simulink model "VK"  (R2022b)
settings: Solver=ode1  StartTime=0.0  StopTime=240  FixedStep=0.01  RelTol=1e-3
undefined symbols (not defined in the file): F, Light, MIL, Newton, Raphson, sigbuilder_block
libraries: simulink x3, aerolibwind2 x2, aerolibutil x1, sharedtransform x1
settings Model: Creator=jmira  LastModifiedBy=armando
settings DebuggingCC: UnconnectedInputMsg=warning  UnconnectedOutputMsg=warning  UnconnectedLineMsg=warning
settings ModelReferenceCC: EnableRefExpFcnMdlSchedulingChecks=on
settings RTWCC: DLArmComputeVersion=19.05

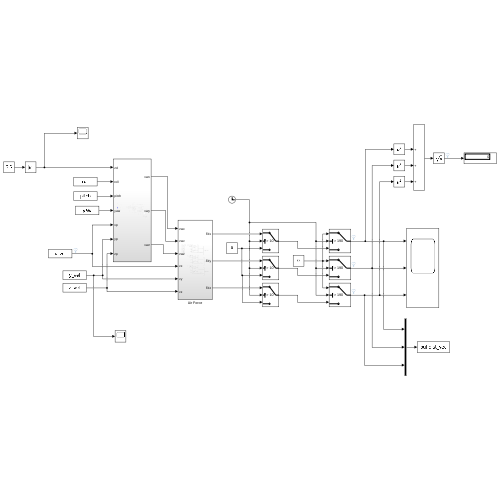
[thumbnail: Simulink's stored preview of the top-level diagram]
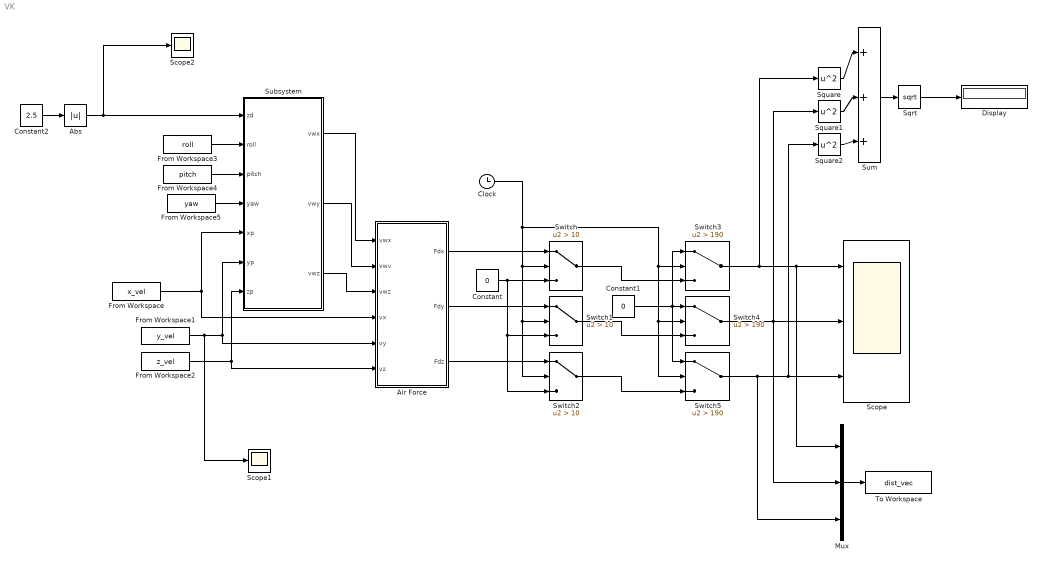
== system VK ==
  Abs : Abs  SaturateOnIntegerOverflow=off
  Air Force : Subsystem
  Clock : Clock
  Constant : Constant  Value=0
  Constant1 : Constant  Value=0
  Constant2 : Constant  Value=2.5
  Display : Display
  From Workspace : FromWorkspace  VariableName=x_vel  SampleTime=0.01
  From Workspace1 : FromWorkspace  VariableName=y_vel  SampleTime=0.01
  From Workspace2 : FromWorkspace  VariableName=z_vel  SampleTime=0.01
  From Workspace3 : FromWorkspace  VariableName=roll  SampleTime=0.01
  From Workspace4 : FromWorkspace  VariableName=pitch  SampleTime=0.01
  From Workspace5 : FromWorkspace  VariableName=yaw  SampleTime=0.01
  Mux : Mux  Inputs=3
  Scope : Scope  NumInputPorts=3
  Scope1 : Scope
  Scope2 : Scope
  Sqrt : Sqrt
  Square : Math  Operator=square
  Square1 : Math  Operator=square
  Square2 : Math  Operator=square
  Subsystem : Subsystem
  Sum : Sum  Inputs=|+++
  Switch : Switch  Criteria=u2 > Threshold  Threshold=10  SaturateOnIntegerOverflow=off  InputSameDT=off
  Switch1 : Switch  Criteria=u2 > Threshold  Threshold=10  SaturateOnIntegerOverflow=off  InputSameDT=off
  Switch2 : Switch  Criteria=u2 > Threshold  Threshold=10  SaturateOnIntegerOverflow=off  InputSameDT=off
  Switch3 : Switch  Criteria=u2 > Threshold  Threshold=190  SaturateOnIntegerOverflow=off  InputSameDT=off
  Switch4 : Switch  Criteria=u2 > Threshold  Threshold=190  SaturateOnIntegerOverflow=off  InputSameDT=off
  Switch5 : Switch  Criteria=u2 > Threshold  Threshold=190  SaturateOnIntegerOverflow=off  InputSameDT=off
  To Workspace : ToWorkspace  VariableName=dist_vec  SampleTime=-1
      settings: Save2DSignal=2-D array (concatenate along first dimension)
  wires:
  Abs/1 -> Scope2/1, Subsystem/1(zd)
  Subsystem/1(vwx) -> Air Force/1(vwx)
  From Workspace/1 -> Air Force/4(vx), Subsystem/5(xp)
  Subsystem/3(vwz) -> Air Force/3(vwz)
  From Workspace1/1 -> Scope1/1, Air Force/5(vy), Subsystem/6(yp)
  Subsystem/2(vwy) -> Air Force/2(vwv)
  From Workspace2/1 -> Air Force/6(vz), Subsystem/7(zp)
  From Workspace3/1 -> Subsystem/2(roll)
  From Workspace4/1 -> Subsystem/3(pitch)
  From Workspace5/1 -> Subsystem/4(yaw)
  Mux/1 -> To Workspace/1
  Air Force/1(Fdx) -> Switch/1
  Clock/1 -> Switch5/2, Switch4/2, Switch3/2, Switch2/2, Switch1/2, Switch/2
  Constant/1 -> Switch2/3, Switch1/3, Switch/3
  Air Force/2(Fdy) -> Switch1/1
  Air Force/3(Fdz) -> Switch2/1
  Switch/1 -> Switch3/3
  Constant1/1 -> Switch5/1, Switch3/1, Switch4/1
  Switch1/1 -> Switch4/3
  Switch2/1 -> Switch5/3
  Switch3/1 -> Square/1, Mux/1, Scope/1
  Switch4/1 -> Square1/1, Mux/2, Scope/2
  Switch5/1 -> Mux/3, Square2/1, Scope/3
  Constant2/1 -> Abs/1
  Square/1 -> Sum/1
  Square2/1 -> Sum/3
  Square1/1 -> Sum/2
  Sum/1 -> Sqrt/1
  Sqrt/1 -> Display/1

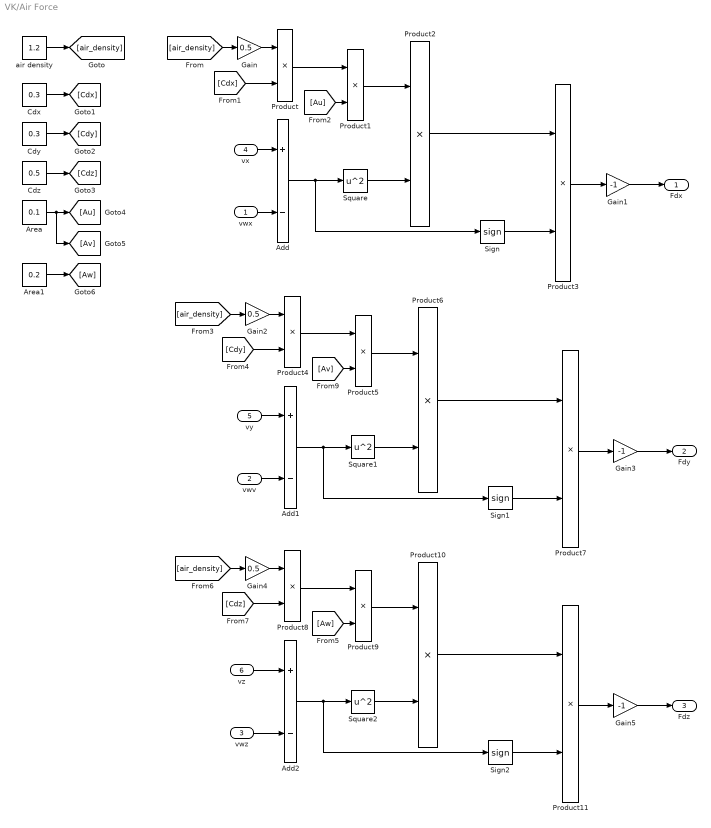
== system VK/Air Force ==
  vwx : Inport
  vwv : Inport  Port=2
  vwz : Inport  Port=3
  vx : Inport  Port=4
  vy : Inport  Port=5
  vz : Inport  Port=6
  Add : Sum  Inputs=+-
  Add1 : Sum  Inputs=+-
  Add2 : Sum  Inputs=+-
  Area : Constant  Value=0.1
  Area1 : Constant  Value=0.2
  Cdx : Constant  Value=0.3
  Cdy : Constant  Value=0.3
  Cdz : Constant  Value=0.5
  Gain : Gain  Gain=0.5
  Gain1 : Gain  Gain=-1
  Gain2 : Gain  Gain=0.5
  Gain3 : Gain  Gain=-1
  Gain4 : Gain  Gain=0.5
  Gain5 : Gain  Gain=-1
  Product{,1..11} (12 alike) : Product
  Sign : Signum
  Sign1 : Signum
  Sign2 : Signum
  Square : Math  Operator=square
  Square1 : Math  Operator=square
  Square2 : Math  Operator=square
  air density : Constant  Value=1.2
  Fdx : Outport
  Fdy : Outport  Port=2
  Fdz : Outport  Port=3
  wires:
  air density/1 -> [air_density]
  [air_density] -> Gain/1
  Cdx/1 -> [Cdx]
  Cdy/1 -> [Cdy]
  Cdz/1 -> [Cdz]
  Gain/1 -> Product/1
  [Cdx] -> Product/2
  Area/1 -> [Av], [Au]
  Product/1 -> Product1/1
  [Au] -> Product1/2
  Product1/1 -> Product2/1
  Square/1 -> Product2/2
  Add/1 -> Sign/1, Square/1
  vx/1 -> Add/1
  vwx/1 -> Add/2
  Product2/1 -> Product3/1
  Sign/1 -> Product3/2
  Product3/1 -> Gain1/1
  Gain1/1 -> Fdx/1
  Gain3/1 -> Fdy/1
  Product7/1 -> Gain3/1
  Sign1/1 -> Product7/2
  Product6/1 -> Product7/1
  vwv/1 -> Add1/2
  vy/1 -> Add1/1
  Add1/1 -> Square1/1, Sign1/1
  Square1/1 -> Product6/2
  Product5/1 -> Product6/1
  [Av] -> Product5/2
  Product4/1 -> Product5/1
  [Cdy] -> Product4/2
  Gain2/1 -> Product4/1
  [air_density] -> Gain2/1
  [air_density] -> Gain4/1
  Gain4/1 -> Product8/1
  [Cdz] -> Product8/2
  Product8/1 -> Product9/1
  [Aw] -> Product9/2
  Product9/1 -> Product10/1
  Square2/1 -> Product10/2
  Add2/1 -> Sign2/1, Square2/1
  Product10/1 -> Product11/1
  Sign2/1 -> Product11/2
  Product11/1 -> Gain5/1
  Gain5/1 -> Fdz/1
  vz/1 -> Add2/1
  vwz/1 -> Add2/2
  Area1/1 -> [Aw]

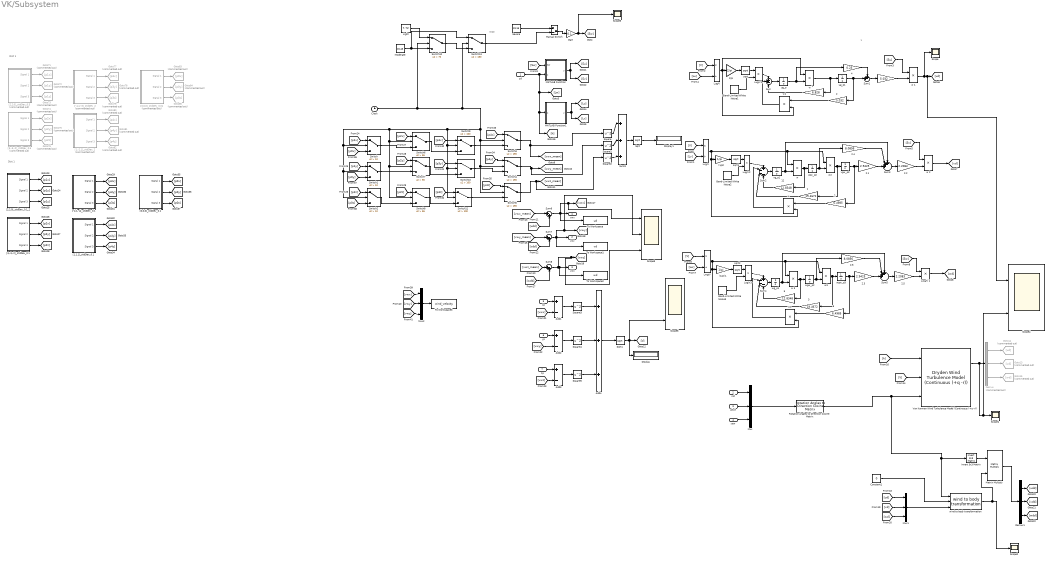
== system VK/Subsystem ==
  note: W20
  note: u
  note: Dist 1
  note: Dist 1
  zd : Inport
  roll : Inport  Port=2
  pitch : Inport  Port=3
  yaw : Inport  Port=4
  xp : Inport  Port=5
  yp : Inport  Port=6
  zp : Inport  Port=7
  " " : Gain  Gain=5.032  SaturateOnIntegerOverflow=on  OutDataTypeStr=Inherit: Same as input  ParamDataTypeStr=Inherit: Same as input
  " 1" : Gain  Gain=6.828  SaturateOnIntegerOverflow=on  OutDataTypeStr=Inherit: Same as input  ParamDataTypeStr=Inherit: Same as input
  " 2" : Gain  Gain=5.032  SaturateOnIntegerOverflow=on  OutDataTypeStr=Inherit: Same as input  ParamDataTypeStr=Inherit: Same as input
  " w" : Product  InputSameDT=on  SaturateOnIntegerOverflow=on  OutDataTypeStr=Inherit: Same as first input
  " w1" : Product  InputSameDT=on  SaturateOnIntegerOverflow=on  OutDataTypeStr=Inherit: Same as first input
  (1/pi) : Gain  Gain=1/pi  SaturateOnIntegerOverflow=on  OutDataTypeStr=Inherit: Same as input  ParamDataTypeStr=Inherit: Same as input
  (1/pi)1 : Gain  Gain=1/pi  SaturateOnIntegerOverflow=on  OutDataTypeStr=Inherit: Same as input  ParamDataTypeStr=Inherit: Same as input
  1 : Gain  Gain=19.4672  SaturateOnIntegerOverflow=on  OutDataTypeStr=Inherit: Same as input  ParamDataTypeStr=Inherit: Same as input
  12 : Gain  Gain=12.8348  SaturateOnIntegerOverflow=on  OutDataTypeStr=Inherit: Same as input  ParamDataTypeStr=Inherit: Same as input
  2 : Gain  Gain=6.4985  SaturateOnIntegerOverflow=on  OutDataTypeStr=Inherit: Same as input  ParamDataTypeStr=Inherit: Same as input
  2.1 : Gain  Gain=2.9425  SaturateOnIntegerOverflow=on  OutDataTypeStr=Inherit: Same as input  ParamDataTypeStr=Inherit: Same as input
  2.2 : Gain  Gain=2.2083  SaturateOnIntegerOverflow=on  OutDataTypeStr=Inherit: Same as input  ParamDataTypeStr=Inherit: Same as input
  2.3 : Gain  Gain=2.9425  SaturateOnIntegerOverflow=on  OutDataTypeStr=Inherit: Same as input  ParamDataTypeStr=Inherit: Same as input
  2.4 : Gain  Gain=8.0856  SaturateOnIntegerOverflow=on  OutDataTypeStr=Inherit: Same as input  ParamDataTypeStr=Inherit: Same as input
  2.5 : Gain  Gain=2.2083  SaturateOnIntegerOverflow=on  OutDataTypeStr=Inherit: Same as input  ParamDataTypeStr=Inherit: Same as input
  2.6 : Gain  Gain=8.0856  SaturateOnIntegerOverflow=on  OutDataTypeStr=Inherit: Same as input  ParamDataTypeStr=Inherit: Same as input
  2/pi : Gain  Gain=2/pi  SaturateOnIntegerOverflow=on  OutDataTypeStr=Inherit: Same as input  ParamDataTypeStr=Inherit: Same as input
  3 : Gain  Gain=19.4672  SaturateOnIntegerOverflow=on  OutDataTypeStr=Inherit: Same as input  ParamDataTypeStr=Inherit: Same as input
  4 : Gain  Gain=0.25  SaturateOnIntegerOverflow=on  OutDataTypeStr=Inherit: Same as input  ParamDataTypeStr=Inherit: Same as input
  5 : Gain  Gain=12.8348  SaturateOnIntegerOverflow=on  OutDataTypeStr=Inherit: Same as input  ParamDataTypeStr=Inherit: Same as input
  6 : Gain  Gain=6.4985  SaturateOnIntegerOverflow=on  OutDataTypeStr=Inherit: Same as input  ParamDataTypeStr=Inherit: Same as input
  Add1 : Sum  Inputs=+-
  Add2 : Sum  Inputs=+-
  Add3 : Sum  Inputs=+-
  Add4 : Sum  Inputs=+++
  Band-Limited White Noise1 : simulink/Sources/Band-Limited White Noise  Cov=3  Ts=0.1  seed=[23341]
  Band-Limited White Noise2 : simulink/Sources/Band-Limited White Noise  Cov=3  Ts=0.1  seed=[23342]
  Band-Limited White Noise3 : simulink/Sources/Band-Limited White Noise  Cov=3  Ts=0.1  seed=[23343]
  Clock : Clock
  Constant1 : Constant  Value=0
  Demux : Demux  Commented=on  Outputs=3
  Demux1 : Demux  Outputs=3
  Display : Display
  Display1 : Display
  Gain : Gain  Gain=0.1
  Goto13 : Goto  Commented=on  GotoTag=vd
  Goto14 : Goto  Commented=on  GotoTag=ud
  Goto15 : Goto  Commented=on  GotoTag=wd
  Goto71 : Goto  Commented=on  GotoTag=p1x
  Goto72 : Goto  Commented=on  GotoTag=p1y
  Goto73 : Goto  Commented=on  GotoTag=p1z
  Goto74 : Goto  Commented=on  GotoTag=p2x
  Goto75 : Goto  Commented=on  GotoTag=p2y
  Goto76 : Goto  Commented=on  GotoTag=p2z
  Goto77 : Goto  Commented=on  GotoTag=p3x
  Goto78 : Goto  Commented=on  GotoTag=p3y
  Goto79 : Goto  Commented=on  GotoTag=p3z
  Goto80 : Goto  Commented=on  GotoTag=p4x
  Goto81 : Goto  Commented=on  GotoTag=p4y
  Goto82 : Goto  Commented=on  GotoTag=p4z
  Goto83 : Goto  Commented=on  GotoTag=p0x
  Goto84 : Goto  Commented=on  GotoTag=p0y
  Goto85 : Goto  Commented=on  GotoTag=p0z
  Invert 3x3 Matrix : aerolibutil/Invert  3x3 Matrix
  Light : Constant  Value=7.72
  Lug/V : Product  Inputs=*/  InputSameDT=on  SaturateOnIntegerOverflow=on  OutDataTypeStr=Inherit: Same as first input
  Lug/V1 : Product  InputSameDT=on  SaturateOnIntegerOverflow=on  OutDataTypeStr=Inherit: Same as first input
  Lug/V2 : Product  InputSameDT=on  SaturateOnIntegerOverflow=on  OutDataTypeStr=Inherit: Same as first input
  Lug/V3 : Product  InputSameDT=on  SaturateOnIntegerOverflow=on  OutDataTypeStr=Inherit: Same as first input
  Lvg/V : Product  Inputs=*/  InputSameDT=on  SaturateOnIntegerOverflow=on  OutDataTypeStr=Inherit: Same as first input
  Lwg/V : Product  Inputs=*/  InputSameDT=on  SaturateOnIntegerOverflow=on  OutDataTypeStr=Inherit: Same as first input
  Lwg/V 1 : Product  InputSameDT=on  SaturateOnIntegerOverflow=on  OutDataTypeStr=Inherit: Same as first input
  MATLAB Function : MATLAB Function  TreatAsAtomicUnit=on
  MATLAB Function1 : MATLAB Function  TreatAsAtomicUnit=on
  Manual Switch : ManualSwitch  CurrentSetting=0
  Matrix Multiply : Product  Multiplication=Matrix(*)
  Moderate : Constant  Value=15.43
  Mux : Mux  Inputs=3
  Mux1 : Mux  Inputs=3
  Mux2 : Mux  Inputs=3
  Rotation Angles to Direction Cosine Matrix : sharedtransform/Rotation Angles to Direction Cosine Matrix  rotationOrder=ZYX  aMode=aMode
  Scope{,1..2,5} (4 alike) : Scope
  Scope3 : Scope  NumInputPorts=3
  Scope4 : Scope  NumInputPorts=2
  Scope6 : Scope  NumInputPorts=3
  Severe : Constant  Value=23.15
  Sqrt : Sqrt
  Sqrt1 : Sqrt
  Square{,1..5} (6 alike) : Math  Operator=square
  Sum : Sum  Inputs=+--  InputSameDT=on  SaturateOnIntegerOverflow=on  OutDataTypeStr=Inherit: Same as first input
  Sum1 : Sum  Inputs=++|  InputSameDT=on  SaturateOnIntegerOverflow=on  OutDataTypeStr=Inherit: Same as first input
  Sum2 : Sum  Inputs=+---  InputSameDT=on  SaturateOnIntegerOverflow=on  OutDataTypeStr=Inherit: Same as first input
  Sum3 : Sum  Inputs=+++||  InputSameDT=on  SaturateOnIntegerOverflow=on  OutDataTypeStr=Inherit: Same as first input
  Sum4 : Sum  Inputs=+---  InputSameDT=on  SaturateOnIntegerOverflow=on  OutDataTypeStr=Inherit: Same as first input
  Sum5 : Sum  Inputs=+++||  InputSameDT=on  SaturateOnIntegerOverflow=on  OutDataTypeStr=Inherit: Same as first input
  Sum6 : Sum  Inputs=|++
  Sum7 : Sum  Inputs=|++
  Sum8 : Sum  Inputs=|++
  Sum9 : Sum  Inputs=|+++
  Switch : Switch  Criteria=u2 > Threshold  Threshold=10  SaturateOnIntegerOverflow=off  InputSameDT=off
  Switch1 : Switch  Criteria=u2 > Threshold  Threshold=10  SaturateOnIntegerOverflow=off  InputSameDT=off
  Switch10 : Switch  Criteria=u2 > Threshold  Threshold=100  SaturateOnIntegerOverflow=off  InputSameDT=off
  Switch11 : Switch  Criteria=u2 > Threshold  Threshold=100  SaturateOnIntegerOverflow=off  InputSameDT=off
  Switch12 : Switch  Criteria=u2 > Threshold  Threshold=70  SaturateOnIntegerOverflow=off  InputSameDT=off
  Switch13 : Switch  Criteria=u2 > Threshold  Threshold=150  SaturateOnIntegerOverflow=off  InputSameDT=off
  Switch2 : Switch  Criteria=u2 > Threshold  Threshold=10  SaturateOnIntegerOverflow=off  InputSameDT=off
  Switch3 : Switch  Criteria=u2 > Threshold  Threshold=155  SaturateOnIntegerOverflow=off  InputSameDT=off
  Switch4 : Switch  Criteria=u2 > Threshold  Threshold=155  SaturateOnIntegerOverflow=off  InputSameDT=off
  Switch5 : Switch  Criteria=u2 > Threshold  Threshold=155  SaturateOnIntegerOverflow=off  InputSameDT=off
  Switch6 : Switch  Criteria=u2 > Threshold  Threshold=55  SaturateOnIntegerOverflow=off  InputSameDT=off
  Switch7 : Switch  Criteria=u2 > Threshold  Threshold=55  SaturateOnIntegerOverflow=off  InputSameDT=off
  Switch8 : Switch  Criteria=u2 > Threshold  Threshold=55  SaturateOnIntegerOverflow=off  InputSameDT=off
  Switch9 : Switch  Criteria=u2 > Threshold  Threshold=100  SaturateOnIntegerOverflow=off  InputSameDT=off
  To Workspace : ToWorkspace  VariableName=ud  SampleTime=-1
      settings: Save2DSignal=2-D array (concatenate along first dimension)
  To Workspace1 : ToWorkspace  VariableName=vd  SampleTime=-1
      settings: Save2DSignal=2-D array (concatenate along first dimension)
  To Workspace2 : ToWorkspace  VariableName=wd  SampleTime=-1
      settings: Save2DSignal=2-D array (concatenate along first dimension)
  To Workspace3 : ToWorkspace  VariableName=wind_velocity  SampleTime=-1
      settings: Save2DSignal=2-D array (concatenate along first dimension)
  Von Karman Wind Turbulence Model (Continuous (+q -r)) : aerolibwind2/Dryden Wind Turbulence Model  (Continuous (+q -r))  units=Metric (MKS)  spec=MIL-F-8785C  model=Continuous Von Karman (+q +r)  W20=15  Wdeg=0  TurbProb=10^-2 - Light  L_high=762  Wingspan=0.5  ts=0.1  Seed=[23341 23342 23343 23344]  T_on=on
  "[-2,1,-4]_stdDev_0.1" : Subsystem  Tag=STV Subsys  LoadFcn=sigbuilder_block('load');  StartFcn=sigbuilder_block('start');  StopFcn=sigbuilder_block('stop');  ClipboardFcn=sigbuilder_block('clipboard');  mask(Sigbuilder block){tuvar=[0:10]}
      mask help: Simulink:masks:SigbuilderBlock_MD
      mask init:
      | if ~strcmp(get_param(bdroot(gcbh),'SimulationStatus'),'stopped') tuvar = sigbuilder_block('maskInit'); end
      settings: CopyFcn=sigbuilder_block('copy');  DeleteFcn=sigbuilder_block('delete');  ModelCloseFcn=sigbuilder_block('modelClose');  PreSaveFcn=sigbuilder_block('preSave');  PauseFcn=sigbuilder_block('pause');  ContinueFcn=sigbuilder_block('continue');  NameChangeFcn=sigbuilder_block('namechange');  OpenFcn=sigbuilder_block('open',[429.75 181.5 550.5 399.75 ]);  CloseFcn=sigbuilder_block('close');
      mask Display: plot(0, 0, 100, 100,[2, 2, 32, 32, 2], [68, 8, 8, 68, 68],[32, 2], [38, 38], [32, 19, 2],[53, 60, 44], [32, 17, 17, 2],[16, 16, 31, 31]);txt = getActiveGroup(gcbh);text(2, 100, txt,'verticalAlignment', 'top');
  "[-4,1,-3]_stdDev_2" : Subsystem  Tag=STV Subsys  Commented=on  LoadFcn=sigbuilder_block('load');  StartFcn=sigbuilder_block('start');  StopFcn=sigbuilder_block('stop');  ClipboardFcn=sigbuilder_block('clipboard');  mask(Sigbuilder block){tuvar=[0:10]}
      mask help: Simulink:masks:SigbuilderBlock_MD
      mask init:
      | if ~strcmp(get_param(bdroot(gcbh),'SimulationStatus'),'stopped') tuvar = sigbuilder_block('maskInit'); end
      settings: CopyFcn=sigbuilder_block('copy');  DeleteFcn=sigbuilder_block('delete');  ModelCloseFcn=sigbuilder_block('modelClose');  PreSaveFcn=sigbuilder_block('preSave');  PauseFcn=sigbuilder_block('pause');  ContinueFcn=sigbuilder_block('continue');  NameChangeFcn=sigbuilder_block('namechange');  OpenFcn=sigbuilder_block('open',[437.6 199.2 550.4 400 ]);  CloseFcn=sigbuilder_block('close');
      mask Display: plot(0, 0, 100, 100,[2, 2, 32, 32, 2], [68, 8, 8, 68, 68],[32, 2], [38, 38], [32, 19, 2],[53, 60, 44], [32, 17, 17, 2],[16, 16, 31, 31]);txt = getActiveGroup(gcbh);text(2, 100, txt,'verticalAlignment', 'top');
  "[0,0,0]_stdDev_0.01" : Subsystem  Tag=STV Subsys  Commented=on  LoadFcn=sigbuilder_block('load');  StartFcn=sigbuilder_block('start');  StopFcn=sigbuilder_block('stop');  ClipboardFcn=sigbuilder_block('clipboard');  mask(Sigbuilder block){tuvar=[0:10]}
      mask help: Simulink:masks:SigbuilderBlock_MD
      mask init:
      | if ~strcmp(get_param(bdroot(gcbh),'SimulationStatus'),'stopped') tuvar = sigbuilder_block('maskInit'); end
      settings: CopyFcn=sigbuilder_block('copy');  DeleteFcn=sigbuilder_block('delete');  ModelCloseFcn=sigbuilder_block('modelClose');  PreSaveFcn=sigbuilder_block('preSave');  PauseFcn=sigbuilder_block('pause');  ContinueFcn=sigbuilder_block('continue');  NameChangeFcn=sigbuilder_block('namechange');  OpenFcn=sigbuilder_block('open',[437.6 199.2 550.4 400 ]);  CloseFcn=sigbuilder_block('close');
      mask Display: plot(0, 0, 100, 100,[2, 2, 32, 32, 2], [68, 8, 8, 68, 68],[32, 2], [38, 38], [32, 19, 2],[53, 60, 44], [32, 17, 17, 2],[16, 16, 31, 31]);txt = getActiveGroup(gcbh);text(2, 100, txt,'verticalAlignment', 'top');
  "[0,0,0]_stdDev_0.1" : Subsystem  Tag=STV Subsys  LoadFcn=sigbuilder_block('load');  StartFcn=sigbuilder_block('start');  StopFcn=sigbuilder_block('stop');  ClipboardFcn=sigbuilder_block('clipboard');  mask(Sigbuilder block){tuvar=[0:10]}
      mask help: Simulink:masks:SigbuilderBlock_MD
      mask init:
      | if ~strcmp(get_param(bdroot(gcbh),'SimulationStatus'),'stopped') tuvar = sigbuilder_block('maskInit'); end
      settings: CopyFcn=sigbuilder_block('copy');  DeleteFcn=sigbuilder_block('delete');  ModelCloseFcn=sigbuilder_block('modelClose');  PreSaveFcn=sigbuilder_block('preSave');  PauseFcn=sigbuilder_block('pause');  ContinueFcn=sigbuilder_block('continue');  NameChangeFcn=sigbuilder_block('namechange');  OpenFcn=sigbuilder_block('open',[437.6 199.2 550.4 400 ]);  CloseFcn=sigbuilder_block('close');
      mask Display: plot(0, 0, 100, 100,[2, 2, 32, 32, 2], [68, 8, 8, 68, 68],[32, 2], [38, 38], [32, 19, 2],[53, 60, 44], [32, 17, 17, 2],[16, 16, 31, 31]);txt = getActiveGroup(gcbh);text(2, 100, txt,'verticalAlignment', 'top');
  "[1,-2,1]_stdDev_2" : Subsystem  Tag=STV Subsys  Commented=on  LoadFcn=sigbuilder_block('load');  StartFcn=sigbuilder_block('start');  StopFcn=sigbuilder_block('stop');  ClipboardFcn=sigbuilder_block('clipboard');  mask(Sigbuilder block){tuvar=[0:10]}
      mask help: Simulink:masks:SigbuilderBlock_MD
      mask init:
      | if ~strcmp(get_param(bdroot(gcbh),'SimulationStatus'),'stopped') tuvar = sigbuilder_block('maskInit'); end
      settings: CopyFcn=sigbuilder_block('copy');  DeleteFcn=sigbuilder_block('delete');  ModelCloseFcn=sigbuilder_block('modelClose');  PreSaveFcn=sigbuilder_block('preSave');  PauseFcn=sigbuilder_block('pause');  ContinueFcn=sigbuilder_block('continue');  NameChangeFcn=sigbuilder_block('namechange');  OpenFcn=sigbuilder_block('open',[437.6 199.2 550.4 400 ]);  CloseFcn=sigbuilder_block('close');
      mask Display: plot(0, 0, 100, 100,[2, 2, 32, 32, 2], [68, 8, 8, 68, 68],[32, 2], [38, 38], [32, 19, 2],[53, 60, 44], [32, 17, 17, 2],[16, 16, 31, 31]);txt = getActiveGroup(gcbh);text(2, 100, txt,'verticalAlignment', 'top');
  "[1,1,1]_stdDev_0.1" : Subsystem  Tag=STV Subsys  LoadFcn=sigbuilder_block('load');  StartFcn=sigbuilder_block('start');  StopFcn=sigbuilder_block('stop');  ClipboardFcn=sigbuilder_block('clipboard');  mask(Sigbuilder block){tuvar=[0:10]}
      mask help: Simulink:masks:SigbuilderBlock_MD
      mask init:
      | if ~strcmp(get_param(bdroot(gcbh),'SimulationStatus'),'stopped') tuvar = sigbuilder_block('maskInit'); end
      settings: CopyFcn=sigbuilder_block('copy');  DeleteFcn=sigbuilder_block('delete');  ModelCloseFcn=sigbuilder_block('modelClose');  PreSaveFcn=sigbuilder_block('preSave');  PauseFcn=sigbuilder_block('pause');  ContinueFcn=sigbuilder_block('continue');  NameChangeFcn=sigbuilder_block('namechange');  OpenFcn=sigbuilder_block('open',[414.75 166.5 580.5 378.75 ]);  CloseFcn=sigbuilder_block('close');
      mask Display: plot(0, 0, 100, 100,[2, 2, 32, 32, 2], [68, 8, 8, 68, 68],[32, 2], [38, 38], [32, 19, 2],[53, 60, 44], [32, 17, 17, 2],[16, 16, 31, 31]);txt = getActiveGroup(gcbh);text(2, 100, txt,'verticalAlignment', 'top');
  "[2,2,0]_stdDev_0.1_2" : Subsystem  Tag=STV Subsys  LoadFcn=sigbuilder_block('load');  StartFcn=sigbuilder_block('start');  StopFcn=sigbuilder_block('stop');  ClipboardFcn=sigbuilder_block('clipboard');  mask(Sigbuilder block){tuvar=[0:10]}
      mask help: Simulink:masks:SigbuilderBlock_MD
      mask init:
      | if ~strcmp(get_param(bdroot(gcbh),'SimulationStatus'),'stopped') tuvar = sigbuilder_block('maskInit'); end
      settings: CopyFcn=sigbuilder_block('copy');  DeleteFcn=sigbuilder_block('delete');  ModelCloseFcn=sigbuilder_block('modelClose');  PreSaveFcn=sigbuilder_block('preSave');  PauseFcn=sigbuilder_block('pause');  ContinueFcn=sigbuilder_block('continue');  NameChangeFcn=sigbuilder_block('namechange');  OpenFcn=sigbuilder_block('open',[684.75 0 558 394.5 ]);  CloseFcn=sigbuilder_block('close');
      mask Display: plot(0, 0, 100, 100,[2, 2, 32, 32, 2], [68, 8, 8, 68, 68],[32, 2], [38, 38], [32, 19, 2],[53, 60, 44], [32, 17, 17, 2],[16, 16, 31, 31]);txt = getActiveGroup(gcbh);text(2, 100, txt,'verticalAlignment', 'top');
  "[2,2,0]_stdDev_0.5" : Subsystem  Tag=STV Subsys  Commented=on  LoadFcn=sigbuilder_block('load');  StartFcn=sigbuilder_block('start');  StopFcn=sigbuilder_block('stop');  ClipboardFcn=sigbuilder_block('clipboard');  mask(Sigbuilder block){tuvar=[0:10]}
      mask help: Simulink:masks:SigbuilderBlock_MD
      mask init:
      | if ~strcmp(get_param(bdroot(gcbh),'SimulationStatus'),'stopped') tuvar = sigbuilder_block('maskInit'); end
      settings: CopyFcn=sigbuilder_block('copy');  DeleteFcn=sigbuilder_block('delete');  ModelCloseFcn=sigbuilder_block('modelClose');  PreSaveFcn=sigbuilder_block('preSave');  PauseFcn=sigbuilder_block('pause');  ContinueFcn=sigbuilder_block('continue');  NameChangeFcn=sigbuilder_block('namechange');  OpenFcn=sigbuilder_block('open',[437.6 199.2 550.4 400 ]);  CloseFcn=sigbuilder_block('close');
      mask Display: plot(0, 0, 100, 100,[2, 2, 32, 32, 2], [68, 8, 8, 68, 68],[32, 2], [38, 38], [32, 19, 2],[53, 60, 44], [32, 17, 17, 2],[16, 16, 31, 31]);txt = getActiveGroup(gcbh);text(2, 100, txt,'verticalAlignment', 'top');
  "[3,-3,-2]_stdDev_0.1" : Subsystem  Tag=STV Subsys  LoadFcn=sigbuilder_block('load');  StartFcn=sigbuilder_block('start');  StopFcn=sigbuilder_block('stop');  ClipboardFcn=sigbuilder_block('clipboard');  mask(Sigbuilder block){tuvar=[0:10]}
      mask help: Simulink:masks:SigbuilderBlock_MD
      mask init:
      | if ~strcmp(get_param(bdroot(gcbh),'SimulationStatus'),'stopped') tuvar = sigbuilder_block('maskInit'); end
      settings: CopyFcn=sigbuilder_block('copy');  DeleteFcn=sigbuilder_block('delete');  ModelCloseFcn=sigbuilder_block('modelClose');  PreSaveFcn=sigbuilder_block('preSave');  PauseFcn=sigbuilder_block('pause');  ContinueFcn=sigbuilder_block('continue');  NameChangeFcn=sigbuilder_block('namechange');  OpenFcn=sigbuilder_block('open',[437.6 200.25 550.4 399.75 ]);  CloseFcn=sigbuilder_block('close');
      mask Display: plot(0, 0, 100, 100,[2, 2, 32, 32, 2], [68, 8, 8, 68, 68],[32, 2], [38, 38], [32, 19, 2],[53, 60, 44], [32, 17, 17, 2],[16, 16, 31, 31]);txt = getActiveGroup(gcbh);text(2, 100, txt,'verticalAlignment', 'top');
  "[3,-3,-2]_stdDev_0.5" : Subsystem  Tag=STV Subsys  Commented=on  LoadFcn=sigbuilder_block('load');  StartFcn=sigbuilder_block('start');  StopFcn=sigbuilder_block('stop');  ClipboardFcn=sigbuilder_block('clipboard');  mask(Sigbuilder block){tuvar=[0:10]}
      mask help: Simulink:masks:SigbuilderBlock_MD
      mask init:
      | if ~strcmp(get_param(bdroot(gcbh),'SimulationStatus'),'stopped') tuvar = sigbuilder_block('maskInit'); end
      settings: CopyFcn=sigbuilder_block('copy');  DeleteFcn=sigbuilder_block('delete');  ModelCloseFcn=sigbuilder_block('modelClose');  PreSaveFcn=sigbuilder_block('preSave');  PauseFcn=sigbuilder_block('pause');  ContinueFcn=sigbuilder_block('continue');  NameChangeFcn=sigbuilder_block('namechange');  OpenFcn=sigbuilder_block('open',[437.6 199.2 550.4 400 ]);  CloseFcn=sigbuilder_block('close');
      mask Display: plot(0, 0, 100, 100,[2, 2, 32, 32, 2], [68, 8, 8, 68, 68],[32, 2], [38, 38], [32, 19, 2],[53, 60, 44], [32, 17, 17, 2],[16, 16, 31, 31]);txt = getActiveGroup(gcbh);text(2, 100, txt,'verticalAlignment', 'top');
  sqrt : Sqrt  AlgorithmType=Newton-Raphson
  sqrt1 : Sqrt  AlgorithmType=Newton-Raphson
  sqrt2 : Sqrt  AlgorithmType=Newton-Raphson
  ug_p : Integrator
  ug_p1 : Integrator
  vg_p1 : Integrator
  vgw_p2 : Integrator
  vgw_p3 : Integrator
  w{,1..3} (4 alike) : Product  InputSameDT=on  SaturateOnIntegerOverflow=on  OutDataTypeStr=Inherit: Same as first input
  w {,1..3} (4 alike) : Product  InputSameDT=on  SaturateOnIntegerOverflow=on  OutDataTypeStr=Inherit: Same as first input
  wg_p1 : Integrator
  wgw_p2 : Integrator
  wgw_p3 : Integrator
  wind to body transformation : aerolibwind2/Dryden Wind Turbulence Model  (Continuous (+q -r))/Select velocities/Low altitude  velocities/wind to body transformation  SystemSampleTime=-1  VariantActivationTime=update diagram  Latency=0  AutoFrameSizeCalculation=off
  vwx : Outport
  vwy : Outport  Port=2
  vwz : Outport  Port=3
  wires:
  [Lu] -> Lug/V/2
  Band-Limited White Noise3/1 -> Lug/V3/2
  Band-Limited White Noise2/1 -> Lug/V2/2
  [Sv] -> w 2/1
  Lug/V2/1 -> Sum2/1
  Lvg/V/1 -> "w "/1, w2/1, (1/pi)/1, " w"/2
  sqrt1/1 -> Lug/V2/1
  vg_p1/1 -> "w "/2, Sum3/1
  (1/pi)/1 -> sqrt1/1
  "w "/1 -> 12/1, vgw_p2/1
  vgw_p2/1 -> w2/2, 2.4/1
  Sum2/1 -> vg_p1/1
  2/1 -> " w"/1
  2.1/1 -> Sum3/3
  2.2/1 -> w 2/2
  Sum3/1 -> 2.2/1
  [Lv] -> Lvg/V/2
  " w"/1 -> Sum2/2
  1/1 -> Sum2/3
  vgw_p3/1 -> 2/1, 2.1/1
  2.4/1 -> Sum3/2
  [Su] -> w 1/1
  ug_p1/1 -> " 2"/1, Sum1/2
  Lug/V/1 -> 2/pi/1, w1/2, w/1
  Band-Limited White Noise1/1 -> Lug/V1/2
  [Sw] -> Lwg/V 1/1
  wg_p1/1 -> w 3/2, Sum5/1
  (1/pi)1/1 -> sqrt2/1
  wgw_p2/1 -> w3/2, 2.6/1
  2/pi/1 -> sqrt/1
  5/1 -> Sum4/4
  Sum5/1 -> 2.5/1
  6/1 -> " w1"/1
  w3/1 -> 3/1, wgw_p3/1
  12/1 -> Sum2/4
  3/1 -> Sum4/3
  wgw_p3/1 -> 6/1, 2.3/1
  " w1"/1 -> Sum4/2
  2.5/1 -> Lwg/V 1/2
  Lug/V1/1 -> Sum/1
  w2/1 -> 1/1, vgw_p3/1
  2.6/1 -> Sum5/2
  ug_p/1 -> 4/1, w/2
  Sum1/1 -> " "/1
  sqrt2/1 -> Lug/V3/1
  Lwg/V/1 -> (1/pi)1/1, " w1"/2, w 3/1, w3/1
  Sum/1 -> ug_p/1
  [Lw] -> Lwg/V/2
  " 2"/1 -> w1/1
  " "/1 -> w 1/2
  w 3/1 -> 5/1, wgw_p2/1
  2.3/1 -> Sum5/3
  sqrt/1 -> Lug/V1/1
  4/1 -> Sum1/1
  " 1"/1 -> Sum/3
  w/1 -> ug_p1/1, " 1"/1
  Sum4/1 -> wg_p1/1
  w1/1 -> Sum/2
  Lug/V3/1 -> Sum4/1
  Gain/1 -> Scope5/1, [Sw]
  [Sw] -> MATLAB Function/1(Sw)
  MATLAB Function/1(y) -> [Sv], [Su]
  MATLAB Function1/1(y) -> [Lv], [Lu]
  Lwg/V 1/1 -> [wd]
  [vwx_mean] -> Sum6/1
  Sum6/1 -> Scope3/1, [vwx], vwx/1, To Workspace/1
  [vwy_mean] -> Sum7/1
  zd/1 -> [h], MATLAB Function1/1(z), [Lw], MATLAB Function/2(z)
  Von Karman Wind Turbulence Model (Continuous (+q -r))/1 -> Scope4/2, Scope1/1, Demux/1
  Demux/1 -> Goto14/1
  Demux/2 -> Goto13/1
  Demux/3 -> Goto15/1
  Mux/1 -> Rotation Angles to Direction Cosine Matrix/1
  roll/1 -> Mux/1
  pitch/1 -> Mux/2
  yaw/1 -> Mux/3
  xp/1 -> Add1/1
  yp/1 -> Add2/1
  zp/1 -> Add3/1
  Add1/1 -> Square3/1
  Add2/1 -> Square4/1
  Add3/1 -> Square5/1
  Square5/1 -> Add4/3
  Square4/1 -> Add4/2
  Square3/1 -> Add4/1
  Sqrt1/1 -> Scope6/3, Display/1, [V]
  [V] -> Lwg/V/1
  [V] -> Lvg/V/1
  [h] -> Von Karman Wind Turbulence Model (Continuous (+q -r))/1
  Add4/1 -> Sqrt1/1
  [vwz_mean] -> Sum8/1
  [wdd] -> Sum8/2
  [vdd] -> Sum7/2
  [udd] -> Sum6/2
  [V] -> Von Karman Wind Turbulence Model (Continuous (+q -r))/2
  Sum7/1 -> [vwy], Scope3/2, To Workspace1/1, vwy/1
  Sum8/1 -> Scope3/3, [vwz], vwz/1, To Workspace2/1
  [V] -> Lug/V/1
  w 1/1 -> Scope/1, Scope4/1, [ud]
  Rotation Angles to Direction Cosine Matrix/1 -> Invert 3x3 Matrix/1, wind to body transformation/1, Von Karman Wind Turbulence Model (Continuous (+q -r))/3
  [ud] -> Mux1/1
  [wd] -> Mux1/3
  Mux1/1 -> wind to body transformation/3
  Constant1/1 -> wind to body transformation/2
  wind to body transformation/1 -> Matrix Multiply/2, Scope2/1
  [vd] -> Mux1/2
  Demux1/1 -> [udd]
  Demux1/2 -> [vdd]
  Demux1/3 -> [wdd]
  w 2/1 -> [vd]
  Invert 3x3 Matrix/1 -> Matrix Multiply/1
  Matrix Multiply/1 -> Demux1/1
  [vwx] -> Add1/2
  [vwy] -> Add2/2
  [vwz] -> Add3/2
  Severe/1 -> Manual Switch/1
  Manual Switch/1 -> Gain/1
  Clock/1 -> Switch12/2, Switch13/2, Switch11/2, Switch10/2, Switch9/2, Switch8/2, Switch7/2, Switch6/2, Switch2/2, Switch1/2, Switch/2, Switch5/2, Switch4/2, Switch3/2
  [p0x] -> Switch/3
  [p0y] -> Switch1/3
  [p0z] -> Switch2/3
  [p4x] -> Switch3/1
  [p4y] -> Switch4/1
  [p4z] -> Switch5/1
  Switch/1 -> Switch6/3
  Switch1/1 -> Switch7/3
  Switch2/1 -> Switch8/3
  Switch9/1 -> Switch3/3
  Switch6/1 -> Switch9/3
  [p3x] -> Switch9/1
  Switch10/1 -> Switch4/3
  Switch7/1 -> Switch10/3
  [p3y] -> Switch10/1
  Switch11/1 -> Switch5/3
  Switch8/1 -> Switch11/3
  [p3z] -> Switch11/1
  [p2x] -> Switch6/1
  [p1x] -> Switch/1
  [p2y] -> Switch7/1
  [p1y] -> Switch1/1
  [p2z] -> Switch8/1
  [p1z] -> Switch2/1
  [vwx] -> Mux2/1
  [vwy] -> Mux2/2
  [vwz] -> Mux2/3
  Mux2/1 -> To Workspace3/1
  "[2,2,0]_stdDev_0.5"/1(Signal 1) -> Goto71/1
  "[2,2,0]_stdDev_0.5"/2(Signal 2) -> Goto72/1
  "[2,2,0]_stdDev_0.5"/3(Signal 3) -> Goto73/1
  "[1,-2,1]_stdDev_2"/3(Signal 3) -> Goto82/1
  "[1,-2,1]_stdDev_2"/2(Signal 2) -> Goto81/1
  "[1,-2,1]_stdDev_2"/1(Signal 1) -> Goto80/1
  "[0,0,0]_stdDev_0.01"/1(Signal 1) -> Goto83/1
  "[0,0,0]_stdDev_0.01"/2(Signal 2) -> Goto84/1
  "[0,0,0]_stdDev_0.01"/3(Signal 3) -> Goto85/1
  "[-4,1,-3]_stdDev_2"/1(Signal 1) -> Goto77/1
  "[-4,1,-3]_stdDev_2"/2(Signal 2) -> Goto78/1
  "[-4,1,-3]_stdDev_2"/3(Signal 3) -> Goto79/1
  "[3,-3,-2]_stdDev_0.5"/1(Signal 1) -> Goto74/1
  "[3,-3,-2]_stdDev_0.5"/2(Signal 2) -> Goto75/1
  "[3,-3,-2]_stdDev_0.5"/3(Signal 3) -> Goto76/1
  "[3,-3,-2]_stdDev_0.1"/3(Signal 3) -> [p2z]
  "[3,-3,-2]_stdDev_0.1"/2(Signal 2) -> [p2y]
  "[3,-3,-2]_stdDev_0.1"/1(Signal 1) -> [p2x]
  "[-2,1,-4]_stdDev_0.1"/3(Signal 3) -> [p3z]
  "[-2,1,-4]_stdDev_0.1"/2(Signal 2) -> [p3y]
  "[-2,1,-4]_stdDev_0.1"/1(Signal 1) -> [p3x]
  "[0,0,0]_stdDev_0.1"/3(Signal 3) -> [p0z]
  "[0,0,0]_stdDev_0.1"/2(Signal 2) -> [p0y]
  "[0,0,0]_stdDev_0.1"/1(Signal 1) -> [p0x]
  "[1,1,1]_stdDev_0.1"/1(Signal 1) -> [p4x]
  "[1,1,1]_stdDev_0.1"/2(Signal 2) -> [p4y]
  "[1,1,1]_stdDev_0.1"/3(Signal 3) -> [p4z]
  "[2,2,0]_stdDev_0.1_2"/3(Signal 3) -> [p1z]
  "[2,2,0]_stdDev_0.1_2"/2(Signal 2) -> [p1y]
  "[2,2,0]_stdDev_0.1_2"/1(Signal 1) -> [p1x]
  Square/1 -> Sum9/1
  Sqrt/1 -> Display1/1
  Switch3/1 -> [vwx_mean], Square/1
  Square2/1 -> Sum9/3
  Switch4/1 -> Square1/1, [vwy_mean]
  Switch5/1 -> Square2/1, [vwz_mean]
  Sum9/1 -> Sqrt/1
  Square1/1 -> Sum9/2
  Switch12/1 -> Switch13/3
  Switch13/1 -> Manual Switch/2
  Light/1 -> Switch12/1
  Moderate/1 -> Switch13/1, Switch12/3

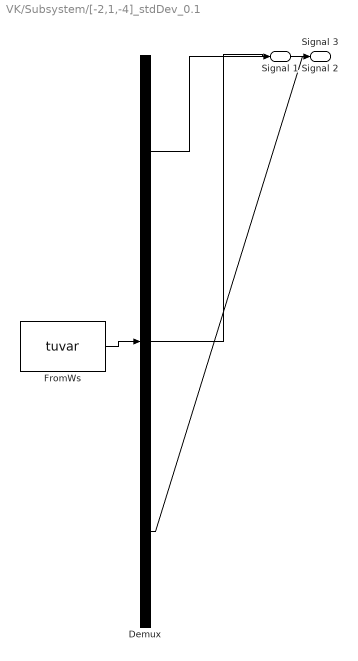
== system VK/Subsystem/[-2,1,-4]_stdDev_0.1 ==
  Demux : Demux  Tag=STV Demux  Outputs=3
      settings: DisplayOption=none
  FromWs : FromWorkspace  Tag=STV FromWs  VariableName=tuvar
      SigBuilderData=|
      | common.afterFinalStr = 'Extrapolate'
      | common.sampleTime = 0
      | dataSet.timeRange = [0 250]
      | dataSet.name = 'Group 1'
      | sbobj.Groups.Name = 'Group 1'
      | sbobj.Groups.Signals(1).Name = 'Signal 1'
      | sbobj.Groups.Signals(1).XData = [0 0.1 0.2 0.3 0.4 0.5 0.6 0.7 0.8 0.9 1 1.1 ... (2501 elements, 1x2501)]
      | sbobj.Groups.Signals(1).YData = [-1.82999016944 -1.95507121864 -1.98781954863 -2.05342964517 -1.86184834588 -1.90961364485 -1.88442841515 -1.73105009614 -1.87061234368 -1.90683276789 -2.04436513758 -2.12458816782 ... (2501 elements, 1x2501)]
      | sbobj.Groups.Signals(2).Name = 'Signal 2'
      | sbobj.Groups.Signals(2).XData = [0 0.1 0.2 0.3 0.4 0.5 0.6 0.7 0.8 0.9 1 1.1 ... (2501 elements, 1x2501)]
      | sbobj.Groups.Signals(2).YData = [0.979334609293 1.02534213584 0.993897740872 0.906106517751 0.986068048139 0.965077359939 1.01724517365 1.04019600767 1.14739273722 0.980026092909 1.00644588389 0.789604529319 ... (2501 elements, 1x2501)]
      | sbobj.Groups.Signals(3).Name = 'Signal 3'
      | sbobj.Groups.Signals(3).XData = [0 0.1 0.2 0.3 0.4 0.5 0.6 0.7 0.8 0.9 1 1.1 ... (2501 elements, 1x2501)]
      | sbobj.Groups.Signals(3).YData = [-4.17480964342 -3.93857727526 -4.07485113678 -4.12458581653 -3.86760422414 -3.95303339354 -3.99481373777 -3.98338227878 -3.83045280443 -4.05187093807 -4.05833878209 -4.16361458885 ... (2501 elements, 1x2501)]
      | sbobj.Groups.TimeRange = [0 250]
  Signal 1 : Outport  Tag=STV Outport
  Signal 2 : Outport  Tag=STV Outport  Port=2
  Signal 3 : Outport  Tag=STV Outport  Port=3
  wires:
  Demux/1 -> Signal 1/1
  FromWs/1 -> Demux/1
  Demux/2 -> Signal 2/1
  Demux/3 -> Signal 3/1

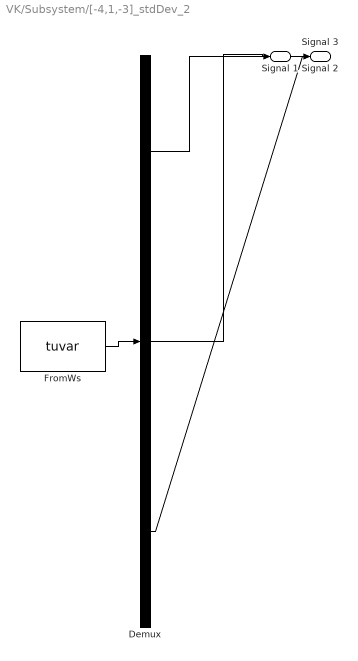
== system VK/Subsystem/[-4,1,-3]_stdDev_2 ==
  Demux : Demux  Tag=STV Demux  Outputs=3
      settings: DisplayOption=none
  FromWs : FromWorkspace  Tag=STV FromWs  VariableName=tuvar
      SigBuilderData=|
      | common.afterFinalStr = 'Extrapolate'
      | common.sampleTime = 0
      | dataSet.timeRange = [0 250]
      | dataSet.name = 'Group 1'
      | sbobj.Groups.Name = 'Group 1'
      | sbobj.Groups.Signals(1).Name = 'Signal 1'
      | sbobj.Groups.Signals(1).XData = [0 0.1 0.2 0.3 0.4 0.5 0.6 0.7 0.8 0.9 1 1.1 ... (2501 elements, 1x2501)]
      | sbobj.Groups.Signals(1).YData = [-3.84543594597 -4.0306848784 -3.88249557229 -4.01419388682 -3.94120508932 -3.98490823082 -4.028485445 -4.09959964476 -3.99990717551 -3.98854277699 -3.995339947 -3.99736823721 ... (2501 elements, 1x2501)]
      | sbobj.Groups.Signals(2).Name = 'Signal 2'
      | sbobj.Groups.Signals(2).XData = [0 0.1 0.2 0.3 0.4 0.5 0.6 0.7 0.8 0.9 1 1.1 ... (2501 elements, 1x2501)]
      | sbobj.Groups.Signals(2).YData = [0.478226810816 0.842826450057 0.957312281117 0.470413435935 1.22425845653 1.01739178181 1.02095388898 1.87598247987 0.253984975139 1.34645377818 1.07472918925 0.631116974138 ... (2501 elements, 1x2501)]
      | sbobj.Groups.Signals(3).Name = 'Signal 3'
      | sbobj.Groups.Signals(3).XData = [0 0.1 0.2 0.3 0.4 0.5 0.6 0.7 0.8 0.9 1 1.1 ... (2501 elements, 1x2501)]
      | sbobj.Groups.Signals(3).YData = [-2.98652934011 -2.82755680021 -2.97206912335 -2.93216545414 -2.83466041098 -2.92241649201 -2.75351214988 -3.1225756868 -3.12600714517 -2.87882236381 -3.04883485037 -2.99465039739 ... (2501 elements, 1x2501)]
      | sbobj.Groups.TimeRange = [0 250]
  Signal 1 : Outport  Tag=STV Outport
  Signal 2 : Outport  Tag=STV Outport  Port=2
  Signal 3 : Outport  Tag=STV Outport  Port=3
  wires:
  Demux/3 -> Signal 3/1
  Demux/2 -> Signal 2/1
  FromWs/1 -> Demux/1
  Demux/1 -> Signal 1/1

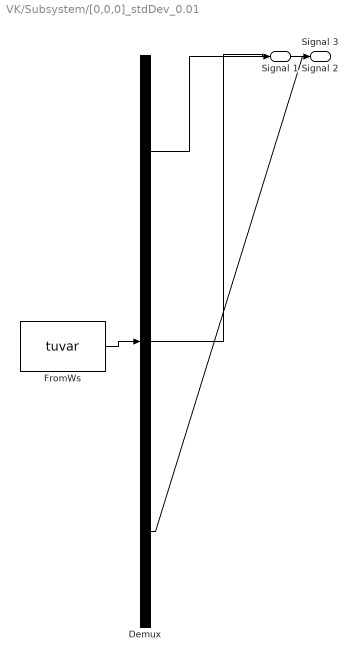
== system VK/Subsystem/[0,0,0]_stdDev_0.01 ==
  Demux : Demux  Tag=STV Demux  Outputs=3
      settings: DisplayOption=none
  FromWs : FromWorkspace  Tag=STV FromWs  VariableName=tuvar
      SigBuilderData=|
      | common.afterFinalStr = 'Extrapolate'
      | common.sampleTime = 0
      | dataSet.timeRange = [0 250]
      | dataSet.name = 'Group 1'
      | sbobj.Groups.Name = 'Group 1'
      | sbobj.Groups.Signals(1).Name = 'Signal 1'
      | sbobj.Groups.Signals(1).XData = [0 0.1 0.2 0.3 0.4 0.5 0.6 0.7 0.8 0.9 1 1.1 ... (2501 elements, 1x2501)]
      | sbobj.Groups.Signals(1).YData = [0.00940144942266 -0.0174346399171 0.0141484583281 -0.00484102254653 0.00527767287347 -0.0117627806114 0.00754808667411 -1.41054873326e-05 0.0125406120773 -0.00546744433677 -0.00735355041208 -0.00756077856404 ... (2501 elements, 1x2501)]
      | sbobj.Groups.Signals(2).Name = 'Signal 2'
      | sbobj.Groups.Signals(2).XData = [0 0.1 0.2 0.3 0.4 0.5 0.6 0.7 0.8 0.9 1 1.1 ... (2501 elements, 1x2501)]
      | sbobj.Groups.Signals(2).YData = [0.00660631387969 0.011571100522 -0.00919389089838 -0.0097052435957 0.00456097775266 -0.0012081562598 0.000128987345423 -0.00885564102881 -0.00948585565674 0.00446796010439 0.0156014644756 -0.00346515774491 ... (2501 elements, 1x2501)]
      | sbobj.Groups.Signals(3).Name = 'Signal 3'
      | sbobj.Groups.Signals(3).XData = [0 0.1 0.2 0.3 0.4 0.5 0.6 0.7 0.8 0.9 1 1.1 ... (2501 elements, 1x2501)]
      | sbobj.Groups.Signals(3).YData = [0.00188414782644 0.00522856248261 0.00504684407057 -0.0142542071699 -0.0020340609317 -0.00240649491107 -0.0234289670646 -0.0131507642934 0.00771962718213 -0.0110061897536 0.0024273740924 -0.0175902685952 ... (2501 elements, 1x2501)]
      | sbobj.Groups.TimeRange = [0 250]
  Signal 1 : Outport  Tag=STV Outport
  Signal 2 : Outport  Tag=STV Outport  Port=2
  Signal 3 : Outport  Tag=STV Outport  Port=3
  wires:
  Demux/1 -> Signal 1/1
  FromWs/1 -> Demux/1
  Demux/2 -> Signal 2/1
  Demux/3 -> Signal 3/1

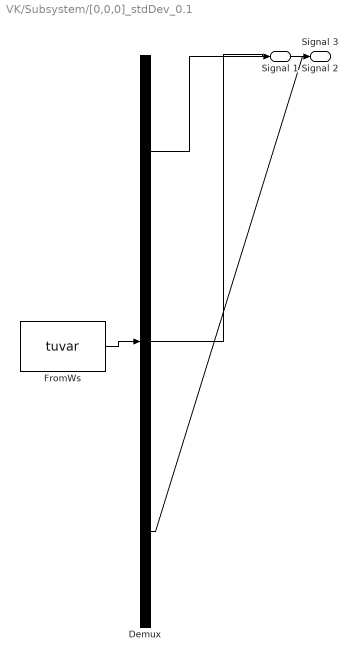
== system VK/Subsystem/[0,0,0]_stdDev_0.1 ==
  Demux : Demux  Tag=STV Demux  Outputs=3
      settings: DisplayOption=none
  FromWs : FromWorkspace  Tag=STV FromWs  VariableName=tuvar
      SigBuilderData=|
      | common.afterFinalStr = 'Extrapolate'
      | common.sampleTime = 0
      | dataSet.timeRange = [0 250]
      | dataSet.name = 'Group 1'
      | sbobj.Groups.Name = 'Group 1'
      | sbobj.Groups.Signals(1).Name = 'Signal 1'
      | sbobj.Groups.Signals(1).XData = [0 0.1 0.2 0.3 0.4 0.5 0.6 0.7 0.8 0.9 1 1.1 ... (2501 elements, 1x2501)]
      | sbobj.Groups.Signals(1).YData = [0.00940144942266 -0.0174346399171 0.0141484583281 -0.00484102254653 0.00527767287347 -0.0117627806114 0.00754808667411 -1.41054873326e-05 0.0125406120773 -0.00546744433677 -0.00735355041208 -0.00756077856404 ... (2501 elements, 1x2501)]
      | sbobj.Groups.Signals(2).Name = 'Signal 2'
      | sbobj.Groups.Signals(2).XData = [0 0.1 0.2 0.3 0.4 0.5 0.6 0.7 0.8 0.9 1 1.1 ... (2501 elements, 1x2501)]
      | sbobj.Groups.Signals(2).YData = [0.00660631387969 0.011571100522 -0.00919389089838 -0.0097052435957 0.00456097775266 -0.0012081562598 0.000128987345423 -0.00885564102881 -0.00948585565674 0.00446796010439 0.0156014644756 -0.00346515774491 ... (2501 elements, 1x2501)]
      | sbobj.Groups.Signals(3).Name = 'Signal 3'
      | sbobj.Groups.Signals(3).XData = [0 0.1 0.2 0.3 0.4 0.5 0.6 0.7 0.8 0.9 1 1.1 ... (2501 elements, 1x2501)]
      | sbobj.Groups.Signals(3).YData = [0.00188414782644 0.00522856248261 0.00504684407057 -0.0142542071699 -0.0020340609317 -0.00240649491107 -0.0234289670646 -0.0131507642934 0.00771962718213 -0.0110061897536 0.0024273740924 -0.0175902685952 ... (2501 elements, 1x2501)]
      | sbobj.Groups.TimeRange = [0 250]
  Signal 1 : Outport  Tag=STV Outport
  Signal 2 : Outport  Tag=STV Outport  Port=2
  Signal 3 : Outport  Tag=STV Outport  Port=3
  wires:
  Demux/3 -> Signal 3/1
  Demux/2 -> Signal 2/1
  FromWs/1 -> Demux/1
  Demux/1 -> Signal 1/1

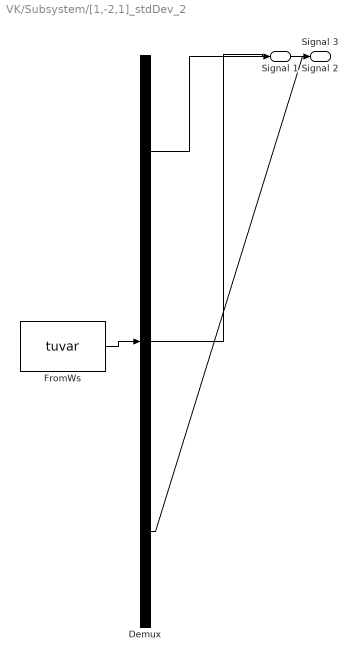
== system VK/Subsystem/[1,-2,1]_stdDev_2 ==
  Demux : Demux  Tag=STV Demux  Outputs=3
      settings: DisplayOption=none
  FromWs : FromWorkspace  Tag=STV FromWs  VariableName=tuvar
      SigBuilderData=|
      | common.afterFinalStr = 'Extrapolate'
      | common.sampleTime = 0
      | dataSet.timeRange = [0 250]
      | dataSet.name = 'Group 1'
      | sbobj.Groups.Name = 'Group 1'
      | sbobj.Groups.Signals(1).Name = 'Signal 1'
      | sbobj.Groups.Signals(1).XData = [0 0.1 0.2 0.3 0.4 0.5 0.6 0.7 0.8 0.9 1 1.1 ... (2501 elements, 1x2501)]
      | sbobj.Groups.Signals(1).YData = [0.75624651904 2.11798505005 1.80071594584 1.10068936755 0.562268392723 0.130668880068 0.754279500324 0.944099462453 0.740001590035 1.2898485583 1.73116128136 1.27973127296 ... (2501 elements, 1x2501)]
      | sbobj.Groups.Signals(2).Name = 'Signal 2'
      | sbobj.Groups.Signals(2).XData = [0 0.1 0.2 0.3 0.4 0.5 0.6 0.7 0.8 0.9 1 1.1 ... (2501 elements, 1x2501)]
      | sbobj.Groups.Signals(2).YData = [-1.83818749097 -2.09440148155 -1.97331014971 -2.58646596302 -1.79615453271 -2.11816846748 -1.30749572887 -1.81270600869 -2.42229273591 -1.5108021506 -1.39738742607 -1.87108536631 ... (2501 elements, 1x2501)]
      | sbobj.Groups.Signals(3).Name = 'Signal 3'
      | sbobj.Groups.Signals(3).XData = [0 0.1 0.2 0.3 0.4 0.5 0.6 0.7 0.8 0.9 1 1.1 ... (2501 elements, 1x2501)]
      | sbobj.Groups.Signals(3).YData = [0.778645690321 0.828921611992 0.810613007202 0.708761800184 1.21087248097 0.996213011829 1.0656983203 0.697614500911 1.99220806301 1.46455723478 1.35215160156 0.940480626562 ... (2501 elements, 1x2501)]
      | sbobj.Groups.TimeRange = [0 250]
  Signal 1 : Outport  Tag=STV Outport
  Signal 2 : Outport  Tag=STV Outport  Port=2
  Signal 3 : Outport  Tag=STV Outport  Port=3
  wires:
  Demux/1 -> Signal 1/1
  FromWs/1 -> Demux/1
  Demux/2 -> Signal 2/1
  Demux/3 -> Signal 3/1

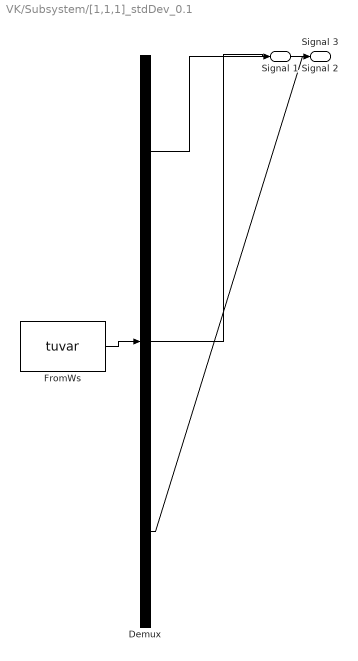
== system VK/Subsystem/[1,1,1]_stdDev_0.1 ==
  Demux : Demux  Tag=STV Demux  Outputs=3
      settings: DisplayOption=none
  FromWs : FromWorkspace  Tag=STV FromWs  VariableName=tuvar
      SigBuilderData=|
      | common.afterFinalStr = 'Extrapolate'
      | common.sampleTime = 0
      | dataSet.timeRange = [0 250]
      | dataSet.name = 'Group 1'
      | sbobj.Groups.Name = 'Group 1'
      | sbobj.Groups.Signals(1).Name = 'Signal 1'
      | sbobj.Groups.Signals(1).XData = [0 0.1 0.2 0.3 0.4 0.5 0.6 0.7 0.8 0.9 1 1.1 ... (2501 elements, 1x2501)]
      | sbobj.Groups.Signals(1).YData = [0.145197088236 -0.0253808832571 0.0817564768307 -0.0799886108636 -0.113716474027 0.0568431012535 -0.140262749373 0.053573846171 0.0401786976598 -0.114921297316 0.150242495944 0.0387933028187 ... (2501 elements, 1x2501)]
      | sbobj.Groups.Signals(2).Name = 'Signal 2'
      | sbobj.Groups.Signals(2).XData = [0 0.1 0.2 0.3 0.4 0.5 0.6 0.7 0.8 0.9 1 1.1 ... (2501 elements, 1x2501)]
      | sbobj.Groups.Signals(2).YData = [0.904254713342 0.977168761781 0.942337679278 0.986229396535 0.809173607241 1.14075260666 0.920222935679 0.898571599624 0.864451326859 0.980227329901 0.977739083111 1.08548184866 ... (2501 elements, 1x2501)]
      | sbobj.Groups.Signals(3).Name = 'Signal 3'
      | sbobj.Groups.Signals(3).XData = [0 0.1 0.2 0.3 0.4 0.5 0.6 0.7 0.8 0.9 1 1.1 ... (2501 elements, 1x2501)]
      | sbobj.Groups.Signals(3).YData = [0.951249303808 1.22359701001 1.16014318917 1.02013787351 0.912453678545 0.826133776014 0.950855900065 0.988819892491 0.948000318007 1.05796971166 1.14623225627 1.05594625459 ... (2501 elements, 1x2501)]
      | sbobj.Groups.TimeRange = [0 250]
  Signal 1 : Outport  Tag=STV Outport
  Signal 2 : Outport  Tag=STV Outport  Port=2
  Signal 3 : Outport  Tag=STV Outport  Port=3
  wires:
  Demux/3 -> Signal 3/1
  Demux/2 -> Signal 2/1
  FromWs/1 -> Demux/1
  Demux/1 -> Signal 1/1

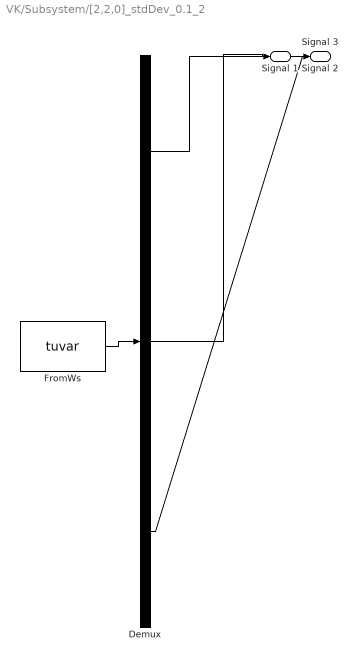
== system VK/Subsystem/[2,2,0]_stdDev_0.1_2 ==
  Demux : Demux  Tag=STV Demux  Outputs=3
      settings: DisplayOption=none
  FromWs : FromWorkspace  Tag=STV FromWs  VariableName=tuvar
      SigBuilderData=|
      | common.afterFinalStr = 'Extrapolate'
      | common.sampleTime = 0
      | dataSet.timeRange = [0 250]
      | dataSet.name = 'Group 1'
      | sbobj.Groups.Name = 'Group 1'
      | sbobj.Groups.Signals(1).Name = 'Signal 1'
      | sbobj.Groups.Signals(1).XData = [0 0.1 0.2 0.3 0.4 0.5 0.6 0.7 0.8 0.9 1 1.1 ... (2501 elements, 1x2501)]
      | sbobj.Groups.Signals(1).YData = [2.03023245951 1.94609273628 1.73805609527 2.05028319058 1.84039968235 2.05480601491 2.03197713458 1.82870042065 2.0243758843 2.13178179015 1.92159752972 1.89506544195 ... (2501 elements, 1x2501)]
      | sbobj.Groups.Signals(2).Name = 'Signal 2'
      | sbobj.Groups.Signals(2).XData = [0 0.1 0.2 0.3 0.4 0.5 0.6 0.7 0.8 0.9 1 1.1 ... (2501 elements, 1x2501)]
      | sbobj.Groups.Signals(2).YData = [1.90426817093 1.98998418636 2.07231920313 1.85041583057 2.0623609141 2.06671706755 2.00438664172 2.1925295132 2.10564241906 1.945520995 1.93382575257 1.92803855073 ... (2501 elements, 1x2501)]
      | sbobj.Groups.Signals(3).Name = 'Signal 3'
      | sbobj.Groups.Signals(3).XData = [0 0.1 0.2 0.3 0.4 0.5 0.6 0.7 0.8 0.9 1 1.1 ... (2501 elements, 1x2501)]
      | sbobj.Groups.Signals(3).YData = [-0.00268027179877 0.068916384047 -0.122578553639 0.198235629235 0.0722139387531 0.0426061788319 -0.106473611766 -0.00208890425378 -0.033586899491 -0.0998438482904 0.187048144588 -0.109383228203 ... (2501 elements, 1x2501)]
      | sbobj.Groups.TimeRange = [0 250]
  Signal 1 : Outport  Tag=STV Outport
  Signal 2 : Outport  Tag=STV Outport  Port=2
  Signal 3 : Outport  Tag=STV Outport  Port=3
  wires:
  Demux/1 -> Signal 1/1
  FromWs/1 -> Demux/1
  Demux/2 -> Signal 2/1
  Demux/3 -> Signal 3/1

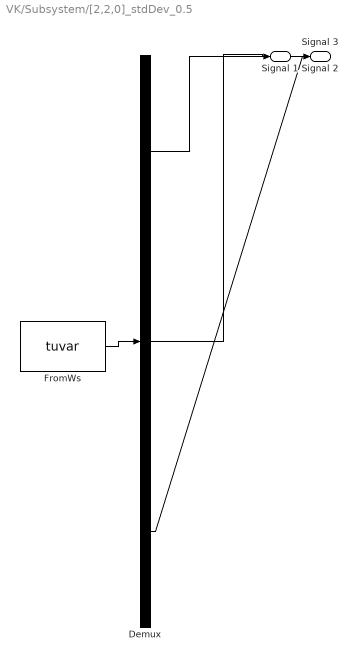
== system VK/Subsystem/[2,2,0]_stdDev_0.5 ==
  Demux : Demux  Tag=STV Demux  Outputs=3
      settings: DisplayOption=none
  FromWs : FromWorkspace  Tag=STV FromWs  VariableName=tuvar
      SigBuilderData=|
      | common.afterFinalStr = 'Extrapolate'
      | common.sampleTime = 0
      | dataSet.timeRange = [0 250]
      | dataSet.name = 'Group 1'
      | sbobj.Groups.Name = 'Group 1'
      | sbobj.Groups.Signals(1).Name = 'Signal 1'
      | sbobj.Groups.Signals(1).XData = [0 0.1 0.2 0.3 0.4 0.5 0.6 0.7 0.8 0.9 1 1.1 ... (2501 elements, 1x2501)]
      | sbobj.Groups.Signals(1).YData = [2.13973814222 2.65410325896 2.47874539465 2.10513444935 2.67670051417 1.94295898568 2.27302777802 1.22311162265 1.38901862914 2.38261307932 1.82294917726 1.79491435889 ... (2501 elements, 1x2501)]
      | sbobj.Groups.Signals(2).Name = 'Signal 2'
      | sbobj.Groups.Signals(2).XData = [0 0.1 0.2 0.3 0.4 0.5 0.6 0.7 0.8 0.9 1 1.1 ... (2501 elements, 1x2501)]
      | sbobj.Groups.Signals(2).YData = [2.0386228398 2.18780372512 2.19778208468 1.94375045552 1.08548164889 3.04572609674 2.1795465611 1.60282762649 1.88634417967 2.79691067744 2.07760281691 2.0892978145 ... (2501 elements, 1x2501)]
      | sbobj.Groups.Signals(3).Name = 'Signal 3'
      | sbobj.Groups.Signals(3).XData = [0 0.1 0.2 0.3 0.4 0.5 0.6 0.7 0.8 0.9 1 1.1 ... (2501 elements, 1x2501)]
      | sbobj.Groups.Signals(3).YData = [0.134299422824 0.512037585052 -0.0168838997908 -1.04539612714 -0.158029639816 0.0664680686666 -0.332514376645 -0.0233756920818 -0.7521221003 -0.336663474628 -0.400204151392 -0.114102499889 ... (2501 elements, 1x2501)]
      | sbobj.Groups.TimeRange = [0 250]
  Signal 1 : Outport  Tag=STV Outport
  Signal 2 : Outport  Tag=STV Outport  Port=2
  Signal 3 : Outport  Tag=STV Outport  Port=3
  wires:
  Demux/3 -> Signal 3/1
  Demux/2 -> Signal 2/1
  FromWs/1 -> Demux/1
  Demux/1 -> Signal 1/1

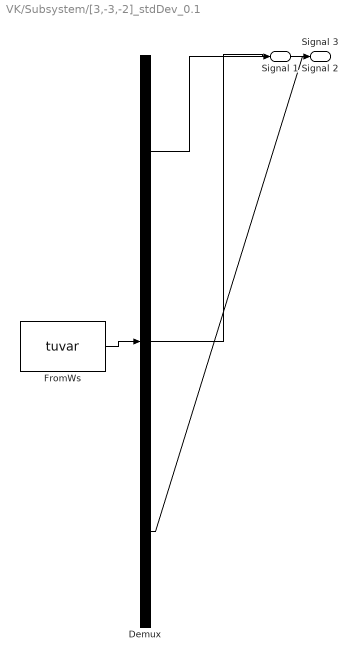
== system VK/Subsystem/[3,-3,-2]_stdDev_0.1 ==
  Demux : Demux  Tag=STV Demux  Outputs=3
      settings: DisplayOption=none
  FromWs : FromWorkspace  Tag=STV FromWs  VariableName=tuvar
      SigBuilderData=|
      | common.afterFinalStr = 'Extrapolate'
      | common.sampleTime = 0
      | dataSet.timeRange = [0 250]
      | dataSet.name = 'Group 1'
      | sbobj.Groups.Name = 'Group 1'
      | sbobj.Groups.Signals(1).Name = 'Signal 1'
      | sbobj.Groups.Signals(1).XData = [0 0.1 0.2 0.3 0.4 0.5 0.6 0.7 0.8 0.9 1 1.1 ... (2501 elements, 1x2501)]
      | sbobj.Groups.Signals(1).YData = [3.09259683816 3.00055104082 2.93655091472 3.08583265349 2.95192235534 3.14897072069 2.93706087935 2.94060492436 2.93713059591 3.03562516496 3.13050857829 3.03656744511 ... (2501 elements, 1x2501)]
      | sbobj.Groups.Signals(2).Name = 'Signal 2'
      | sbobj.Groups.Signals(2).XData = [0 0.1 0.2 0.3 0.4 0.5 0.6 0.7 0.8 0.9 1 1.1 ... (2501 elements, 1x2501)]
      | sbobj.Groups.Signals(2).YData = [-1.56596473413 -1.81811002648 -2.73124905974 -2.43186795963 -2.13749981027 -1.79917024722 -2.65137300533 -1.82893995085 -2.43755865019 -2.67797298424 -1.78096638523 -1.44739190299 ... (2501 elements, 1x2501)]
      | sbobj.Groups.Signals(3).Name = 'Signal 3'
      | sbobj.Groups.Signals(3).XData = [0 0.1 0.2 0.3 0.4 0.5 0.6 0.7 0.8 0.9 1 1.1 ... (2501 elements, 1x2501)]
      | sbobj.Groups.Signals(3).YData = [-0.901663395159 -1.16163865593 -1.13281205685 -1.34780016913 -1.17989469592 0.154359912458 -0.0809779707473 -0.473295261845 -0.82961598066 -0.251639604636 -1.21475605525 -1.86148332625 ... (2501 elements, 1x2501)]
      | sbobj.Groups.TimeRange = [0 250]
  Signal 1 : Outport  Tag=STV Outport
  Signal 2 : Outport  Tag=STV Outport  Port=2
  Signal 3 : Outport  Tag=STV Outport  Port=3
  wires:
  Demux/3 -> Signal 3/1
  Demux/2 -> Signal 2/1
  FromWs/1 -> Demux/1
  Demux/1 -> Signal 1/1

== system VK/Subsystem/[3,-3,-2]_stdDev_0.5 ==
  Demux : Demux  Tag=STV Demux  Outputs=3
      settings: DisplayOption=none
  FromWs : FromWorkspace  Tag=STV FromWs  VariableName=tuvar
      SigBuilderData=|
      | common.afterFinalStr = 'Extrapolate'
      | common.sampleTime = 0
      | dataSet.timeRange = [0 250]
      | dataSet.name = 'Group 1'
      | sbobj.Groups.Name = 'Group 1'
      | sbobj.Groups.Signals(1).Name = 'Signal 1'
      | sbobj.Groups.Signals(1).XData = [0 0.1 0.2 0.3 0.4 0.5 0.6 0.7 0.8 0.9 1 1.1 ... (2501 elements, 1x2501)]
      | sbobj.Groups.Signals(1).YData = [3.26883356977 3.9169425073 1.8705765695 3.43108666018 3.15938261993 2.34615585185 2.78320398885 3.17131223327 4.78919846986 4.38471851494 2.32505652992 4.51746173317 ... (2501 elements, 1x2501)]
      | sbobj.Groups.Signals(2).Name = 'Signal 2'
      | sbobj.Groups.Signals(2).XData = [0 0.1 0.2 0.3 0.4 0.5 0.6 0.7 0.8 0.9 1 1.1 ... (2501 elements, 1x2501)]
      | sbobj.Groups.Signals(2).YData = [-2.97528267623 -2.46097706259 -2.84591062001 -2.85018072865 -3.09860922777 -3.07321121647 -3.05153543489 -4.39949097292 -2.80336241198 -2.50487642367 -3.64881645534 -3.76098418102 ... (2501 elements, 1x2501)]
      | sbobj.Groups.Signals(3).Name = 'Signal 3'
      | sbobj.Groups.Signals(3).XData = [0 0.1 0.2 0.3 0.4 0.5 0.6 0.7 0.8 0.9 1 1.1 ... (2501 elements, 1x2501)]
      | sbobj.Groups.Signals(3).YData = [-1.53701580921 -1.99724479588 -2.3172454264 -1.57083673256 -2.2403882233 -1.25514639654 -2.31469560327 -2.2969753782 -2.31434702043 -1.8218741752 -1.34745710857 -1.81716277443 ... (2501 elements, 1x2501)]
      | sbobj.Groups.TimeRange = [0 250]
  Signal 1 : Outport  Tag=STV Outport
  Signal 2 : Outport  Tag=STV Outport  Port=2
  Signal 3 : Outport  Tag=STV Outport  Port=3
  wires:
  Demux/1 -> Signal 1/1
  FromWs/1 -> Demux/1
  Demux/2 -> Signal 2/1
  Demux/3 -> Signal 3/1

== matlab function VK/Subsystem/MATLAB Function1 ==
  data: y output; z input
function y = fcn(z)

y = z/((0.177 + 0.000823*z)^1.2);

== matlab function VK/Subsystem/MATLAB Function ==
  data: Sw input; y output; z input
function y = fcn(Sw,z)

y = Sw/((0.177 + 0.000823*z)^0.4);
